simulink model "mpc_no_load"  (R2020a)
settings: Solver=FixedStepAuto  StartTime=0.0  StopTime=sim_time  RelTol=1e-3
InitFcn:
  | ros_init_callback
values from neighbouring files (symbols this model uses):
  Ts_mpc = Ts    [initialize_mpc_iris_no_load.m]    (also in initialize_mpc_iris_payload.m)
  Ts_pos_control = 0.01    [initialise_ros_iris_payload.m]
  Ts_sub = 0.01    [initialise_ros_iris_payload.m]
undefined symbols (not defined in the file or in its folder): AccelerationOrForce, enable_mpc, mpc_start_time, TypeMask, use_mpc_control, Yaw
libraries: robotlib x9, simulink x3, robotgazebolib x1
settings Model: Creator=esl  LastModifiedBy=mluser
settings DebuggingCC: SFMachineParentedDataDiag=error

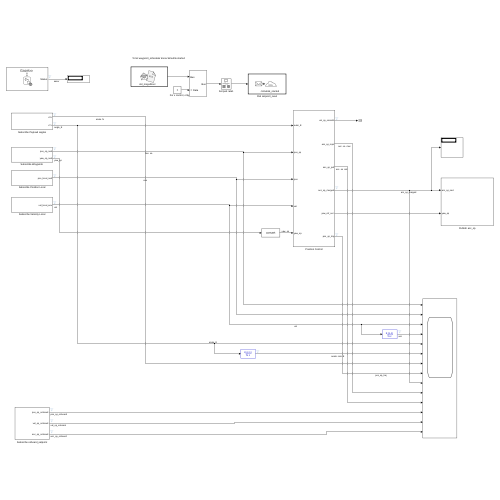
[thumbnail: Simulink's stored preview of the top-level diagram]
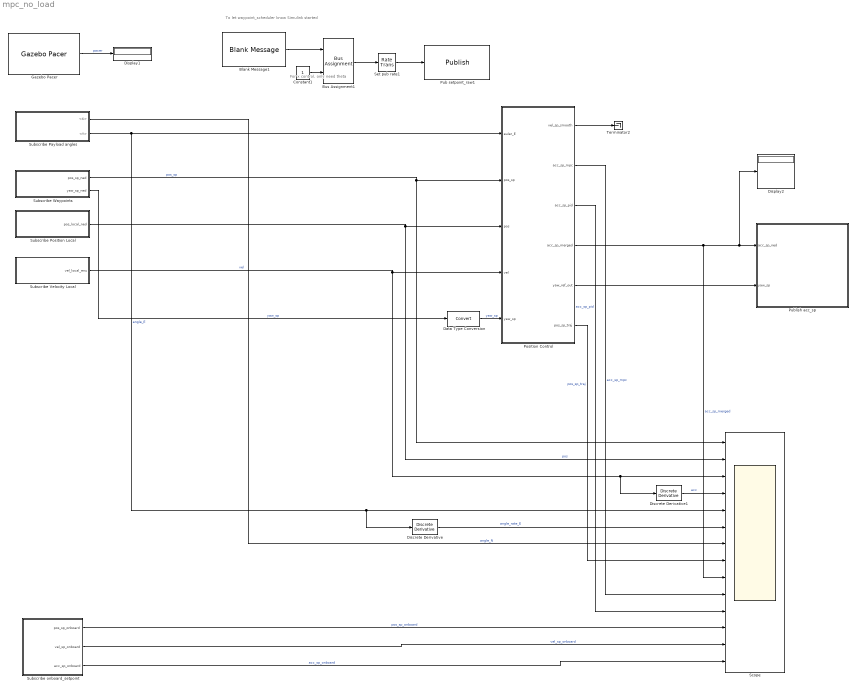
== system mpc_no_load ==
  note: For x control, only need theta
  note: To let waypoint_scheduler know Simulink started
  Blank Message1 : robotlib/Blank Message  messageClass=Message  entityType=std_msgs/Bool  messageType=std_msgs/Bool  SampleTime=inf  legacyBusStruct=off
  Bus Assignment1 : BusAssignment  AssignedSignals=Data
  Constant1 : Constant  OutDataTypeStr=boolean
  Data Type Conversion : DataTypeConversion
  Discrete Derivative : simulink/Discrete/Discrete Derivative  gainval=1.0  ICPrevScaledInput=0.0  OutMin=[]  OutMax=[]  OutDataType=fixdt(1, 16)  OutScaling=2^-10  DoSatur=off
  Discrete Derivative1 : simulink/Discrete/Discrete Derivative  gainval=1.0  ICPrevScaledInput=0.0  OutMin=[]  OutMax=[]  OutDataType=fixdt(1, 16)  OutScaling=2^-10  DoSatur=off
  Display1 : Display
  Display2 : Display
  Gazebo Pacer : robotgazebolib/Gazebo Pacer  ResetBehavior=Reset Gazebo simulation time  SampleTime=0.004
      settings: SourceProductBaseCode=RO
  Position Control : Subsystem
  Pub setpoint_raw1 : robotlib/Publish  topicSource=Specify your own  topic=/simulink_started  messageType=std_msgs/Bool  legacyBusStruct=off  messageQueueLength=1
  Publish acc_sp : Subsystem
  Scope : Scope  NumInputPorts=14
  Set pub rate1 : RateTransition  OutPortSampleTime=Ts_pub_setpoint
  Subscribe Payload angles : Subsystem
  Subscribe Position Local : Subsystem
  Subscribe Velocity Local : Subsystem
  Subscribe Waypoints : Subsystem
  Subscribe onboard_setpoint : Subsystem
  Terminator2 : Terminator
  wires:
  Subscribe Position Local/1(pos_local_ned) -> Scope/2, Position Control/3(pos)  "pos"
  Subscribe Waypoints/1(pos_sp_ned) -> Scope/1, Position Control/2(pos_sp)  "pos_sp"
  Gazebo Pacer/1 -> Display1/1  "pacer"
  Data Type Conversion/1 -> Position Control/5(yaw_sp)  "yaw_sp"
  Subscribe Waypoints/2(yaw_sp_ned) -> Data Type Conversion/1  "yaw_sp"
  Position Control/4(acc_sp_merged) -> Scope/9, Display2/1, Publish acc_sp/1(acc_sp_ned)  "acc_sp_merged"
  Blank Message1/1 -> Bus Assignment1/1
  Constant1/1 -> Bus Assignment1/2
  Bus Assignment1/1 -> Set pub rate1/1
  Set pub rate1/1 -> Pub setpoint_raw1/1
  Subscribe Velocity Local/1(vel_local_enu) -> Scope/3, Discrete Derivative1/1, Position Control/4(vel)  "vel"
  Position Control/5("yaw_ref_out ") -> Publish acc_sp/2(yaw_sp)
  Position Control/1(vel_sp_smooth) -> Terminator2/1
  Position Control/2(acc_sp_mpc) -> Scope/10  "acc_sp_mpc"
  Position Control/3(acc_sp_pid) -> Scope/11  "acc_sp_pid"
  Subscribe onboard_setpoint/3(acc_sp_onboard) -> Scope/14  "acc_sp_onboard"
  Subscribe onboard_setpoint/2(vel_sp_onboard) -> Scope/13  "vel_sp_onboard"
  Subscribe onboard_setpoint/1(pos_sp_onboard) -> Scope/12  "pos_sp_onboard"
  Subscribe Payload angles/1(<X>) -> Scope/7  "angle_N"
  Discrete Derivative/1 -> Scope/6  "angle_rate_E"
  Subscribe Payload angles/2(<Y>) -> Discrete Derivative/1, Scope/5, Position Control/1(euler_E)  "angle_E"
  Position Control/6(pos_sp_traj) -> Scope/8  "pos_sp_traj"
  Discrete Derivative1/1 -> Scope/4  "acc"

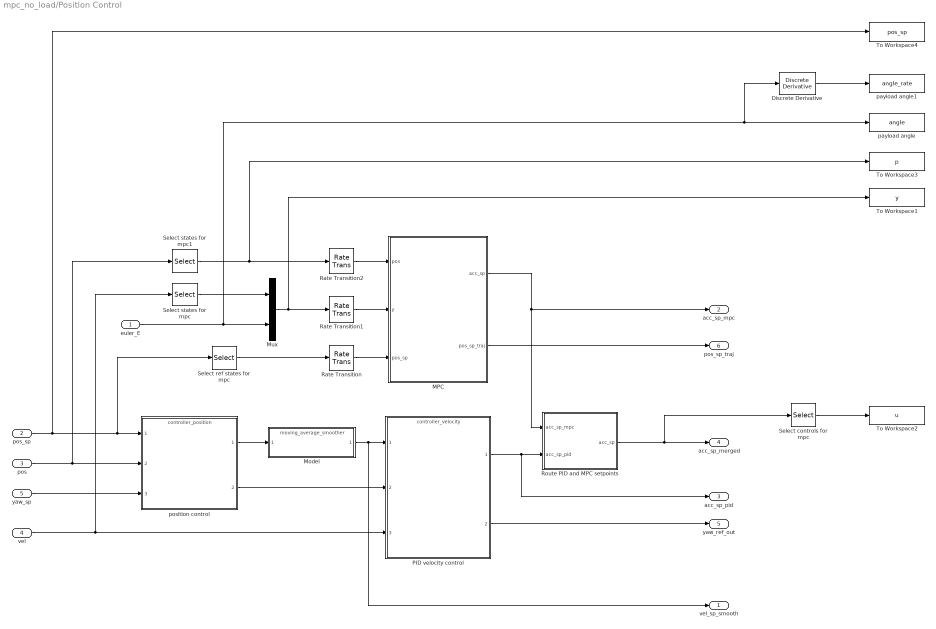
== system mpc_no_load/Position Control ==
  euler_E : Inport  SampleTime=Ts_pos_control
  pos_sp : Inport  Port=2
  pos : Inport  Port=3
  vel : Inport  Port=4
  yaw_sp : Inport  Port=5
  Discrete Derivative : simulink/Discrete/Discrete Derivative  gainval=1.0  ICPrevScaledInput=0.0  OutMin=[]  OutMax=[]  OutDataType=fixdt(1, 16)  OutScaling=2^-10  DoSatur=off
  MPC : Subsystem  Variant=on  AllowZeroVariantControls=on
  Model : ModelReference  ModelNameDialog=moving_average_smoother.slx  SimulationMode=Normal  ModelReferenceVersion=1.4
  Mux : Mux  Inputs=2
  PID velocity control : ModelReference  ModelNameDialog=controller_velocity.slx  SimulationMode=Normal  ModelReferenceVersion=3.10
  Rate Transition : RateTransition  Deterministic=off  OutPortSampleTime=Ts_mpc
  Rate Transition1 : RateTransition  Deterministic=off  OutPortSampleTime=Ts_mpc
  Rate Transition2 : RateTransition  Deterministic=off
  Route PID and MPC setpoints : Subsystem
  Select controls for mpc : Selector  InputPortWidth=3  IndexOptions=Index vector (dialog)  Indices=mpc_states  OutputSizes=1
  Select ref states for mpc : Selector  InputPortWidth=3  IndexOptions=Index vector (dialog)  Indices=mpc_states  OutputSizes=1
  Select states for mpc : Selector  InputPortWidth=3  IndexOptions=Index vector (dialog)  Indices=mpc_states  OutputSizes=1
  Select states for mpc1 : Selector  InputPortWidth=3  IndexOptions=Index vector (dialog)  Indices=mpc_states  OutputSizes=1
  To Workspace1 : ToWorkspace  VariableName=y  SaveFormat=Timeseries  SampleTime=Ts_pos_control
  To Workspace2 : ToWorkspace  VariableName=u  SaveFormat=Timeseries  SampleTime=Ts_pos_control
  To Workspace3 : ToWorkspace  VariableName=p  SaveFormat=Timeseries  SampleTime=Ts_pos_control
  To Workspace4 : ToWorkspace  VariableName=pos_sp  SaveFormat=Timeseries  SampleTime=Ts_pos_control
  payload angle : ToWorkspace  VariableName=angle  SaveFormat=Timeseries  SampleTime=Ts_pos_control
  payload angle1 : ToWorkspace  VariableName=angle_rate  SaveFormat=Timeseries  SampleTime=Ts_mpc
  position control : ModelReference  ModelNameDialog=controller_position.slx  SimulationMode=Normal  ModelReferenceVersion=4.12
  vel_sp_smooth : Outport
  acc_sp_mpc : Outport  Port=2
  acc_sp_pid : Outport  Port=3
  acc_sp_merged : Outport  Port=4
  "yaw_ref_out " : Outport  Port=5
  pos_sp_traj : Outport  Port=6  OutDataTypeStr=double  PortDimensions=nu
  wires:
  PID velocity control/2 -> "yaw_ref_out "/1
  Rate Transition2/1 -> MPC/1(pos)
  Rate Transition1/1 -> MPC/2(y)
  Mux/1 -> Rate Transition1/1, To Workspace1/1
  yaw_sp/1 -> position control/3
  MPC/1(acc_sp) -> acc_sp_mpc/1, Route PID and MPC setpoints/1(acc_sp_mpc)
  Select states for mpc/1 -> Mux/1
  vel/1 -> Select states for mpc/1, PID velocity control/3
  Rate Transition/1 -> MPC/3(pos_sp)
  Route PID and MPC setpoints/1(acc_sp) -> acc_sp_merged/1, Select controls for mpc/1
  position control/2 -> PID velocity control/2
  PID velocity control/1 -> acc_sp_pid/1, Route PID and MPC setpoints/2(acc_sp_pid)
  pos_sp/1 -> To Workspace4/1, Select ref states for mpc/1, position control/1
  Select controls for mpc/1 -> To Workspace2/1
  pos/1 -> Select states for mpc1/1, position control/2
  Select ref states for mpc/1 -> Rate Transition/1
  position control/1 -> Model/1
  Model/1 -> vel_sp_smooth/1, PID velocity control/1
  Select states for mpc1/1 -> To Workspace3/1, Rate Transition2/1
  euler_E/1 -> Mux/2, Discrete Derivative/1, payload angle/1
  Discrete Derivative/1 -> payload angle1/1
  MPC/2(pos_sp_traj) -> pos_sp_traj/1

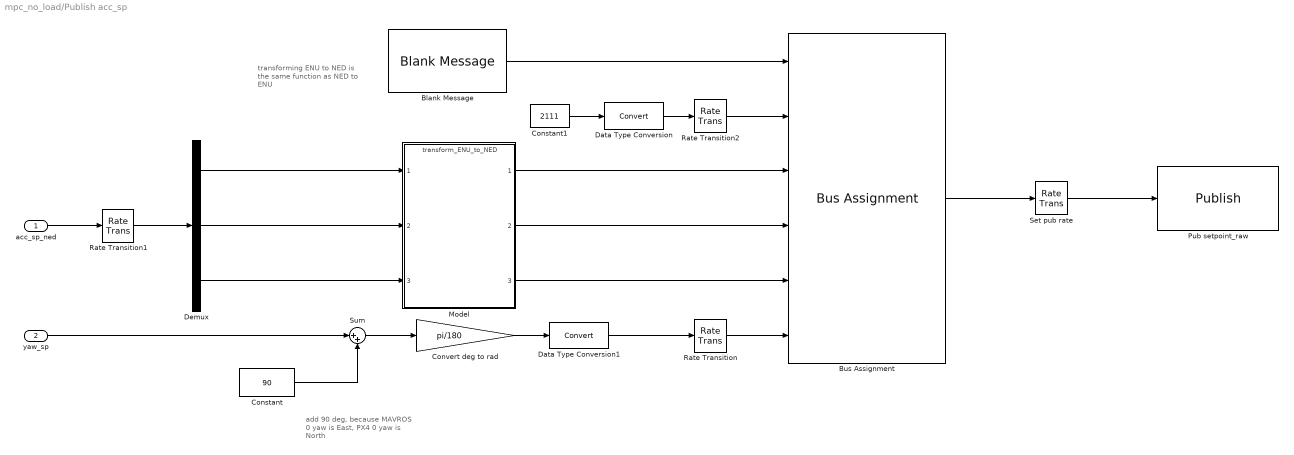
== system mpc_no_load/Publish acc_sp ==
  note: add 90 deg, because
      | MAVROS 0 yaw is East,
      | PX4 0 yaw is North
  note: transforming
      | ENU to NED
      | is the same function as
      | NED to ENU
  acc_sp_ned : Inport
  yaw_sp : Inport  Port=2
  Blank Message : robotlib/Blank Message  messageClass=Message  entityType=mavros_msgs/PositionTarget  messageType=mavros_msgs/PositionTarget  SampleTime=inf  legacyBusStruct=off
  Bus Assignment : BusAssignment  AssignedSignals=TypeMask,AccelerationOrForce.X,AccelerationOrForce.Y,AccelerationOrForce.Z,Yaw
  Constant : Constant  Value=90
  Constant1 : Constant  Value=2111
  Convert deg to rad : Gain  Gain=pi/180
  Data Type Conversion : DataTypeConversion
  Data Type Conversion1 : DataTypeConversion
  Demux : Demux  Outputs=3
  Model : ModelReference  ModelNameDialog=transform_ENU_to_NED.slx  SimulationMode=Normal  ModelReferenceVersion=1.10
  Pub setpoint_raw : robotlib/Publish  topicSource=Select from ROS network  topic=/mavros/setpoint_raw/local  messageType=mavros_msgs/PositionTarget  legacyBusStruct=off  messageQueueLength=1
  Rate Transition : RateTransition  OutPortSampleTimeOpt=Inherit  OutPortSampleTime=0.03
  Rate Transition1 : RateTransition  OutPortSampleTimeOpt=Inherit
  Rate Transition2 : RateTransition  OutPortSampleTimeOpt=Inherit
  Set pub rate : RateTransition  OutPortSampleTime=Ts_pub_setpoint
  Sum : Sum  Inputs=|++
  wires:
  Data Type Conversion/1 -> Rate Transition2/1
  Sum/1 -> Convert deg to rad/1
  Rate Transition/1 -> Bus Assignment/6
  acc_sp_ned/1 -> Rate Transition1/1
  Constant1/1 -> Data Type Conversion/1
  yaw_sp/1 -> Sum/1
  Blank Message/1 -> Bus Assignment/1
  Rate Transition2/1 -> Bus Assignment/2
  Bus Assignment/1 -> Set pub rate/1
  Rate Transition1/1 -> Demux/1
  Constant/1 -> Sum/2
  Set pub rate/1 -> Pub setpoint_raw/1
  Data Type Conversion1/1 -> Rate Transition/1
  Demux/1 -> Model/1
  Demux/2 -> Model/2
  Demux/3 -> Model/3
  Model/1 -> Bus Assignment/3
  Model/2 -> Bus Assignment/4
  Model/3 -> Bus Assignment/5
  Convert deg to rad/1 -> Data Type Conversion1/1

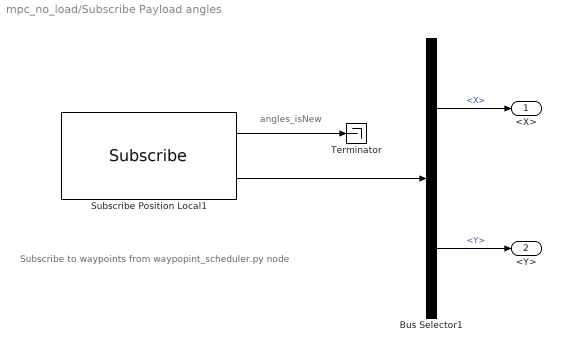
== system mpc_no_load/Subscribe Payload angles ==
  note: angles_isNew
  note: Subscribe to waypoints from waypopint_scheduler.py node
  Bus Selector1 : BusSelector  OutputSignals=X,Y
  Subscribe Position Local1 : robotlib/Subscribe  topicSource=Select from ROS network  topic=/payload_angles_local  messageType=geometry_msgs/Vector3  SampleTime=Ts_sub  legacyBusStruct=off  messageQueueLength=1
  Terminator : Terminator
  <X> : Outport
  <Y> : Outport  Port=2
  wires:
  Subscribe Position Local1/1 -> Terminator/1
  Subscribe Position Local1/2 -> Bus Selector1/1
  Bus Selector1/2 -> <Y>/1  "<Y>"
  Bus Selector1/1 -> <X>/1  "<X>"

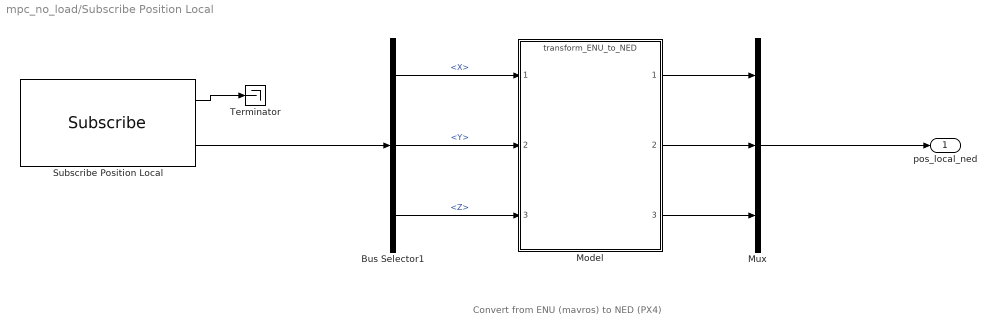
== system mpc_no_load/Subscribe Position Local ==
  note: Convert from ENU (mavros) to NED (PX4)
  Bus Selector1 : BusSelector  OutputSignals=Pose.Position.X,Pose.Position.Y,Pose.Position.Z
  Model : ModelReference  ModelNameDialog=transform_ENU_to_NED.slx  SimulationMode=Normal  ModelReferenceVersion=1.10
  Mux : Mux  Inputs=3
  Subscribe Position Local : robotlib/Subscribe  topicSource=Select from ROS network  topic=/mavros/local_position/pose  messageType=geometry_msgs/PoseStamped  SampleTime=Ts_sub  legacyBusStruct=off  messageQueueLength=1
  Terminator : Terminator
  pos_local_ned : Outport
  wires:
  Subscribe Position Local/1 -> Terminator/1
  Mux/1 -> pos_local_ned/1
  Subscribe Position Local/2 -> Bus Selector1/1
  Bus Selector1/1 -> Model/1  "<X>"
  Bus Selector1/2 -> Model/2  "<Y>"
  Bus Selector1/3 -> Model/3  "<Z>"
  Model/1 -> Mux/1
  Model/2 -> Mux/2
  Model/3 -> Mux/3

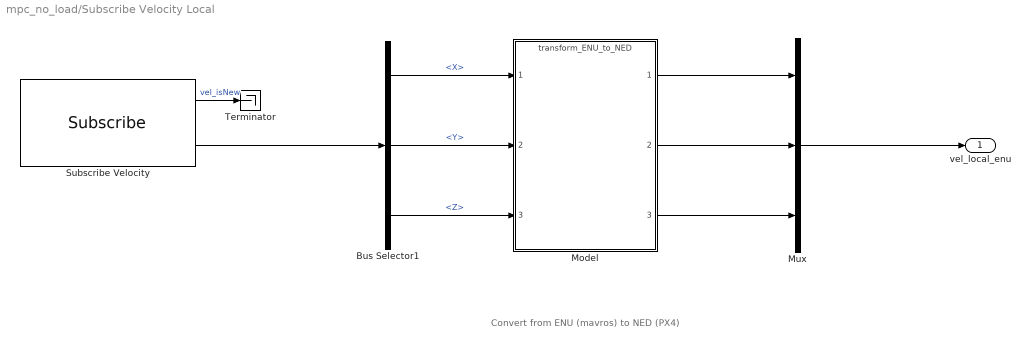
== system mpc_no_load/Subscribe Velocity Local ==
  note: Convert from ENU (mavros) to NED (PX4)
  Bus Selector1 : BusSelector  OutputSignals=Twist.Linear.X,Twist.Linear.Y,Twist.Linear.Z
  Model : ModelReference  ModelNameDialog=transform_ENU_to_NED.slx  SimulationMode=Normal  ModelReferenceVersion=1.10
  Mux : Mux  Inputs=3
  Subscribe Velocity : robotlib/Subscribe  topicSource=Select from ROS network  topic=/mavros/local_position/velocity_local  messageType=geometry_msgs/TwistStamped  SampleTime=Ts_sub  legacyBusStruct=off  messageQueueLength=1
  Terminator : Terminator
  vel_local_enu : Outport
  wires:
  Subscribe Velocity/1 -> Terminator/1  "vel_isNew"
  Subscribe Velocity/2 -> Bus Selector1/1
  Mux/1 -> vel_local_enu/1
  Bus Selector1/1 -> Model/1  "<X>"
  Bus Selector1/2 -> Model/2  "<Y>"
  Bus Selector1/3 -> Model/3  "<Z>"
  Model/1 -> Mux/1
  Model/2 -> Mux/2
  Model/3 -> Mux/3

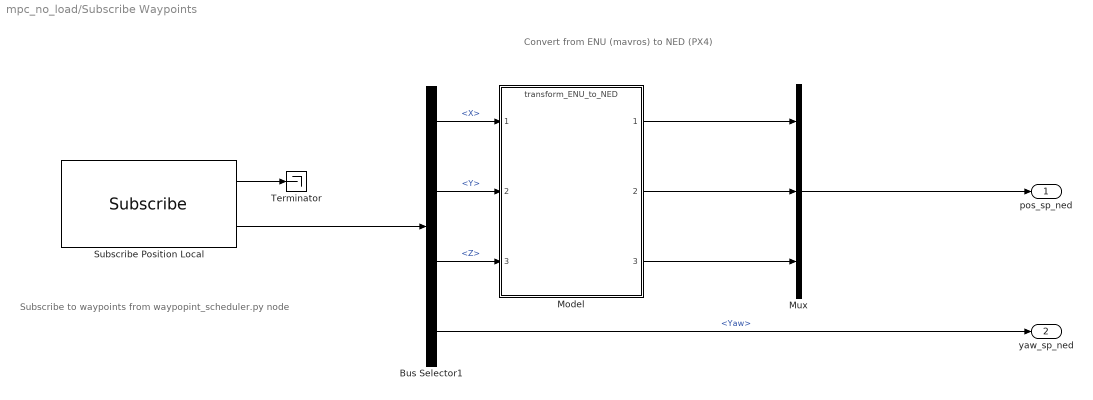
== system mpc_no_load/Subscribe Waypoints ==
  note: Subscribe to waypoints from waypopint_scheduler.py node
  note: Convert from ENU (mavros) to NED (PX4)
  Bus Selector1 : BusSelector  OutputSignals=Position.X,Position.Y,Position.Z,Yaw
  Model : ModelReference  ModelNameDialog=transform_ENU_to_NED.slx  SimulationMode=Normal  ModelReferenceVersion=1.10
  Mux : Mux  Inputs=3
  Subscribe Position Local : robotlib/Subscribe  topicSource=Select from ROS network  topic=/setpoint_raw/local  messageType=mavros_msgs/PositionTarget  SampleTime=Ts_sub  legacyBusStruct=off  messageQueueLength=1
  Terminator : Terminator
  pos_sp_ned : Outport
  yaw_sp_ned : Outport  Port=2
  wires:
  Subscribe Position Local/1 -> Terminator/1
  Subscribe Position Local/2 -> Bus Selector1/1
  Bus Selector1/4 -> yaw_sp_ned/1  "<Yaw>"
  Mux/1 -> pos_sp_ned/1
  Bus Selector1/1 -> Model/1  "<X>"
  Bus Selector1/2 -> Model/2  "<Y>"
  Bus Selector1/3 -> Model/3  "<Z>"
  Model/1 -> Mux/1
  Model/2 -> Mux/2
  Model/3 -> Mux/3

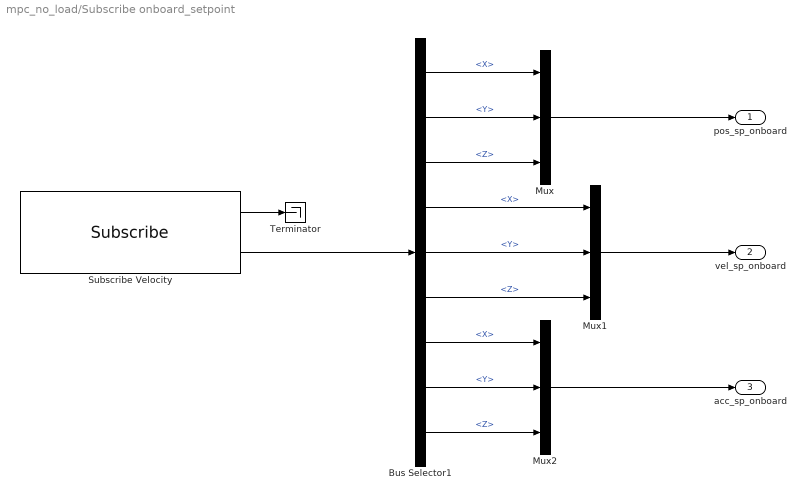
== system mpc_no_load/Subscribe onboard_setpoint ==
  Bus Selector1 : BusSelector  OutputSignals=Position.X,Position.Y,Position.Z,Velocity.X,Velocity.Y,Velocity.Z,AccelerationOrForce.X,AccelerationOrForce.Y,AccelerationOrForce.Z
  Mux : Mux  Inputs=3
  Mux1 : Mux  Inputs=3
  Mux2 : Mux  Inputs=3
  Subscribe Velocity : robotlib/Subscribe  topicSource=Select from ROS network  topic=/mavros/setpoint_raw/target_local  messageType=mavros_msgs/PositionTarget  SampleTime=Ts_sub  legacyBusStruct=off  messageQueueLength=1
  Terminator : Terminator
  pos_sp_onboard : Outport
  vel_sp_onboard : Outport  Port=2
  acc_sp_onboard : Outport  Port=3
  wires:
  Subscribe Velocity/1 -> Terminator/1
  Subscribe Velocity/2 -> Bus Selector1/1
  Mux/1 -> pos_sp_onboard/1
  Bus Selector1/1 -> Mux/1  "<X>"
  Bus Selector1/2 -> Mux/2  "<Y>"
  Bus Selector1/3 -> Mux/3  "<Z>"
  Mux1/1 -> vel_sp_onboard/1
  Bus Selector1/4 -> Mux1/1  "<X>"
  Bus Selector1/5 -> Mux1/2  "<Y>"
  Bus Selector1/6 -> Mux1/3  "<Z>"
  Bus Selector1/8 -> Mux2/2  "<Y>"
  Bus Selector1/7 -> Mux2/1  "<X>"
  Bus Selector1/9 -> Mux2/3  "<Z>"
  Mux2/1 -> acc_sp_onboard/1

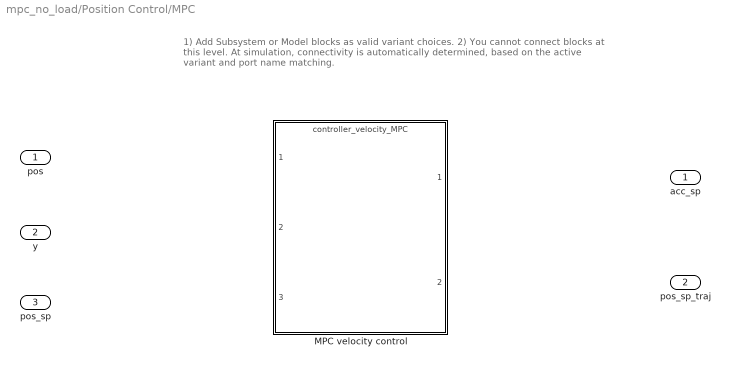
== system mpc_no_load/Position Control/MPC ==
  note: 1) Add Subsystem or Model blocks as valid variant choices.
      | 2) You cannot connect blocks at this level. At simulation, connectivity is automatically
      | determined, based on the active variant and port name matching.
  pos : Inport  OutDataTypeStr=double  SampleTime=Ts_mpc
  y : Inport  Port=2  OutDataTypeStr=double  SampleTime=Ts_mpc
  pos_sp : Inport  Port=3  OutDataTypeStr=double  SampleTime=Ts_mpc
  MPC velocity control : ModelReference  ModelNameDialog=controller_velocity_MPC.slx  SimulationMode=Normal  VariantControl=mpc_variant  ModelReferenceVersion=3.50
  acc_sp : Outport  OutDataTypeStr=double  PortDimensions=nu
  pos_sp_traj : Outport  Port=2  OutDataTypeStr=double  PortDimensions=nu

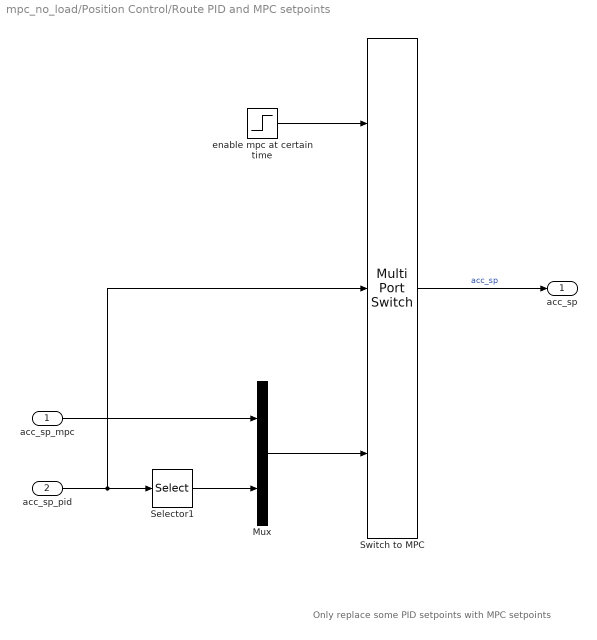
== system mpc_no_load/Position Control/Route PID and MPC setpoints ==
  note: Only replace some PID setpoints with MPC setpoints
  acc_sp_mpc : Inport
  acc_sp_pid : Inport  Port=2  PortDimensions=3
  Mux : Mux  Inputs=2
  Selector1 : Selector  InputPortWidth=3  IndexOptions=Index vector (dialog)  Indices=pid_states  OutputSizes=1
  Switch to MPC : MultiPortSwitch  DataPortOrder=Zero-based contiguous  Inputs=2  zeroidx=on
  enable mpc at certain time : Step  Time=mpc_start_time  After=enable_mpc*use_mpc_control  SampleTime=0
  acc_sp : Outport  PortDimensions=3
  wires:
  enable mpc at certain time/1 -> Switch to MPC/1
  acc_sp_pid/1 -> Switch to MPC/2, Selector1/1
  acc_sp_mpc/1 -> Mux/1
  Selector1/1 -> Mux/2
  Mux/1 -> Switch to MPC/3
  Switch to MPC/1 -> acc_sp/1  "acc_sp"
